simulink model "ThreatMAV"  (R2026a)
settings: Solver=VariableStepAuto
undefined symbols (not defined in the file): CrashCmd, spoofTime, ts_uav
libraries: uavmavlinklib x2
settings Model: DataDictionary=QuadData.sldd  Creator=The MathWorks, Inc.  LastModifiedBy=The MathWorks, Inc.

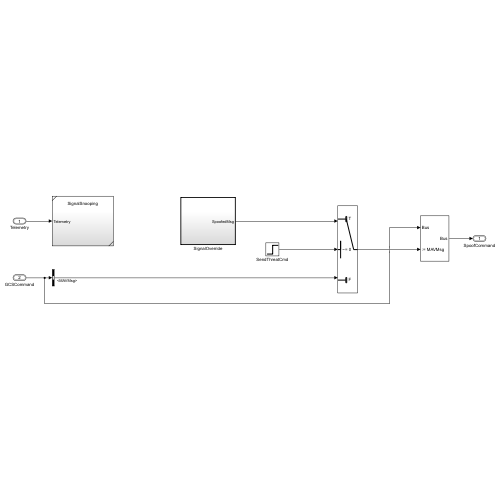
[thumbnail: Simulink's stored preview of the top-level diagram]
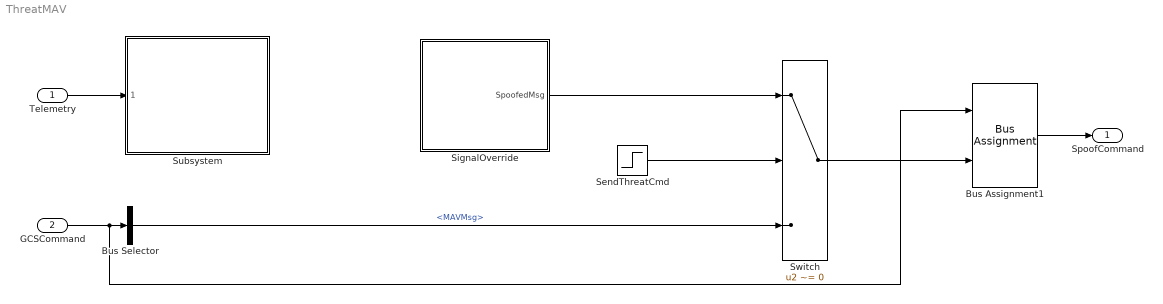
== system ThreatMAV ==
  Telemetry : Inport  OutDataTypeStr=Bus: Telemetry  SampleTime=ts_uav
  GCSCommand : Inport  Port=2  OutDataTypeStr=Bus: GCSCmds  SampleTime=ts_uav  BusOutputAsStruct=on
  Bus Assignment1 : BusAssignment  AssignedSignals=MAVMsg
  Bus Selector : BusSelector  OutputSignals=MAVMsg
  SendThreatCmd : Step  Time=spoofTime  SampleTime=ts_uav
  SignalOverride : Subsystem  TreatAsAtomicUnit=on
  Subsystem : Subsystem  ReferencedSubsystem=SignalSnooping
  Switch : Switch  Criteria=u2 ~= 0  SaturateOnIntegerOverflow=off  InputSameDT=off
  SpoofCommand : Outport  OutDataTypeStr=Bus: GCSCmds  BusOutputAsStruct=on
  wires:
  GCSCommand/1 -> Bus Assignment1/1, Bus Selector/1
  SignalOverride/1(SpoofedMsg) -> Switch/1
  SendThreatCmd/1 -> Switch/2
  Bus Assignment1/1 -> SpoofCommand/1
  Switch/1 -> Bus Assignment1/2
  Bus Selector/1 -> Switch/3  "<MAVMsg>"
  Telemetry/1 -> Subsystem/1

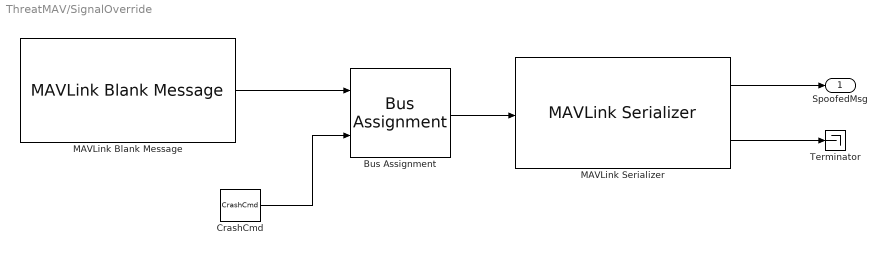
== system ThreatMAV/SignalOverride ==
  Bus Assignment : BusAssignment  AssignedSignals=Payload.base_mode
  CrashCmd : Constant  Value=CrashCmd  OutDataTypeStr=uint8
  MAVLink Blank Message : uavmavlinklib/MAVLink Blank Message  dialectSource=Select from standard MAVLink dialects  dialect=common.xml  dialectCustom=common.xml  version=2  messageType=SET_MODE  SystemID=1  ComponentID=1  SampleTime=-1
  MAVLink Serializer : uavmavlinklib/MAVLink Serializer  dialectSource=Select from standard MAVLink dialects  dialect=common.xml  dialectCustom=common.xml  version=2  messageType=SET_MODE
  Terminator : Terminator
  SpoofedMsg : Outport
  wires:
  Bus Assignment/1 -> MAVLink Serializer/1
  CrashCmd/1 -> Bus Assignment/2
  MAVLink Blank Message/1 -> Bus Assignment/1
  MAVLink Serializer/2 -> Terminator/1
  MAVLink Serializer/1 -> SpoofedMsg/1
